simulink model "desacoplamento"  (Simulink 7.1)
settings: Solver=ode45  StartTime=0.0  StopTime=10.0  RelTol=1e-3
values from neighbouring files (symbols this model uses):
  A = [-4  0  -2; 0  -4  1; 2.66666666667  -2.66666666667  0]    [lab 06.mat]
  AA = [0  1  0; 0  0  1; -32  -24  -8]    [lab 06.mat]
  B = [2 0 0]    [lab 06.mat]
  BB = [0 0 21.3333333333]    [lab 06.mat]
  D = [0 0 0 0]    [lab 06.mat]
  r1 = 2    [lab 06.mat]
  r2 = 4    [lab 06.mat]
settings Model: Creator=ALUNO  LastModifiedBy=ALUNO

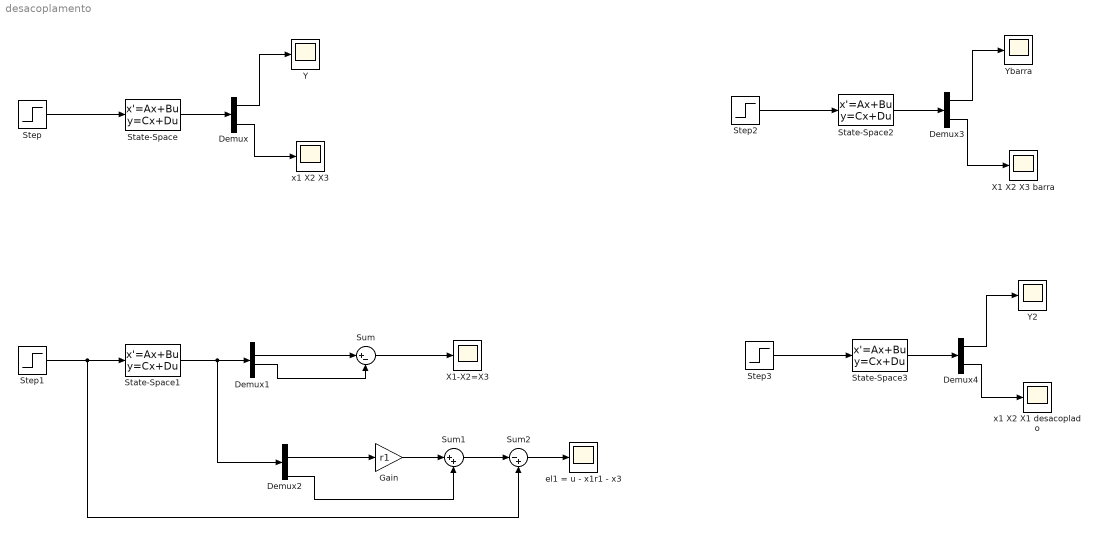
== system desacoplamento ==
  Demux : Demux  Outputs=[1 3]
  Demux1 : Demux
  Demux2 : Demux
  Demux3 : Demux  Outputs=[1 3]
  Demux4 : Demux  Outputs=[1 3]
  Gain : Gain  Gain=r1  ParameterDataType=sfix(16)  ParameterScaling=2^0  OutDataType=sfix(16)  OutScaling=2^0
  State-Space : StateSpace  A=A  B=B  C=[0 r2 0;1 0 0;0 1 0;0 0 1]  D=D
  State-Space1 : StateSpace  A=A  B=B  C=[0 r2 0;1 0 0;0 1 0;0 0 1]  D=D
  State-Space2 : StateSpace  A=AA  B=BB  C=[0 r2 0;1 0 0;0 1 0;0 0 1]  D=D
  State-Space3 : StateSpace  A=A  B=B  C=[0 r2 0;1 0 0;0 1 0;0 0 1]  D=D
  Step{,1..3} (4 alike) : Step  SampleTime=0
  Sum : Sum  Inputs=|+-  OutDataType=sfix(16)  OutScaling=2^0
  Sum1 : Sum  Inputs=|++  OutDataType=sfix(16)  OutScaling=2^0
  Sum2 : Sum  Inputs=|-+  OutDataType=sfix(16)  OutScaling=2^0
  X1 X2 X3 barra : Scope
      settings: SaveName=ScopeData5
  X1-X2=X3 : Scope
      settings: SaveName=ScopeData3
  Y : Scope
  Y2 : Scope
      settings: SaveName=ScopeData6
  Ybarra : Scope
      settings: SaveName=ScopeData4
  el1 = u - x1r1 - x3 : Scope
      settings: SaveName=ScopeData2
  x1 X2 X1 desacoplado : Scope
      settings: SaveName=ScopeData7
  x1 X2 X3 : Scope
  wires:
  Step/1 -> State-Space/1
  State-Space/1 -> Demux/1
  Demux/1 -> Y/1
  Demux/2 -> x1 X2 X3/1
  Step1/1 -> State-Space1/1, Sum2/2
  State-Space1/1 -> Demux1/1, Demux2/1
  Demux1/2 -> Sum/1
  Demux1/3 -> Sum/2
  Sum/1 -> X1-X2=X3/1
  Gain/1 -> Sum1/1
  Demux2/2 -> Gain/1
  Demux2/4 -> Sum1/2
  Sum1/1 -> Sum2/1
  Sum2/1 -> el1 = u - x1r1 - x3/1
  Step2/1 -> State-Space2/1
  State-Space2/1 -> Demux3/1
  Demux3/1 -> Ybarra/1
  Demux3/2 -> X1 X2 X3 barra/1
  Step3/1 -> State-Space3/1
  State-Space3/1 -> Demux4/1
  Demux4/1 -> Y2/1
  Demux4/2 -> x1 X2 X1 desacoplado/1
